simulink model "CoproductReact"  (R2023b)
settings: Solver=VariableStepAuto  StartTime=0.0  StopTime=10.0  RelTol=1e-3
values from neighbouring files (symbols this model uses):
  sug_init = 1011.832    [init_4_sim.m]    (also in init_sim.m = 1011; init_sim2.m; init_sim_suggarferm.m)
  volume = 25    [init_4_sim.m]    (also in init_sim.m; init_sim2.m; init_sim_suggarferm.m)
  yeast_gram = 11    [init_4_sim.m]    (also in init_sim2.m; init_sim_suggarferm.m)
settings Model: Creator=20181234  LastModifiedBy=20181234

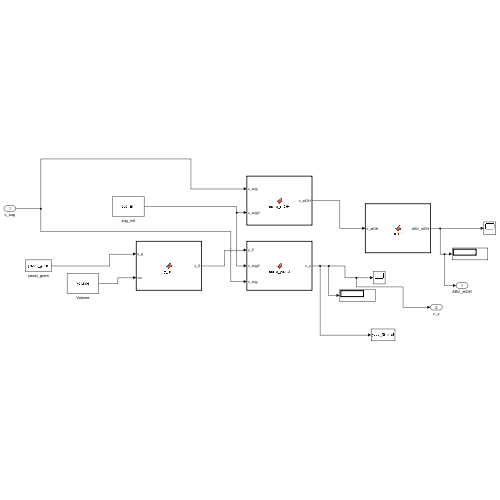
[thumbnail: Simulink's stored preview of the top-level diagram]
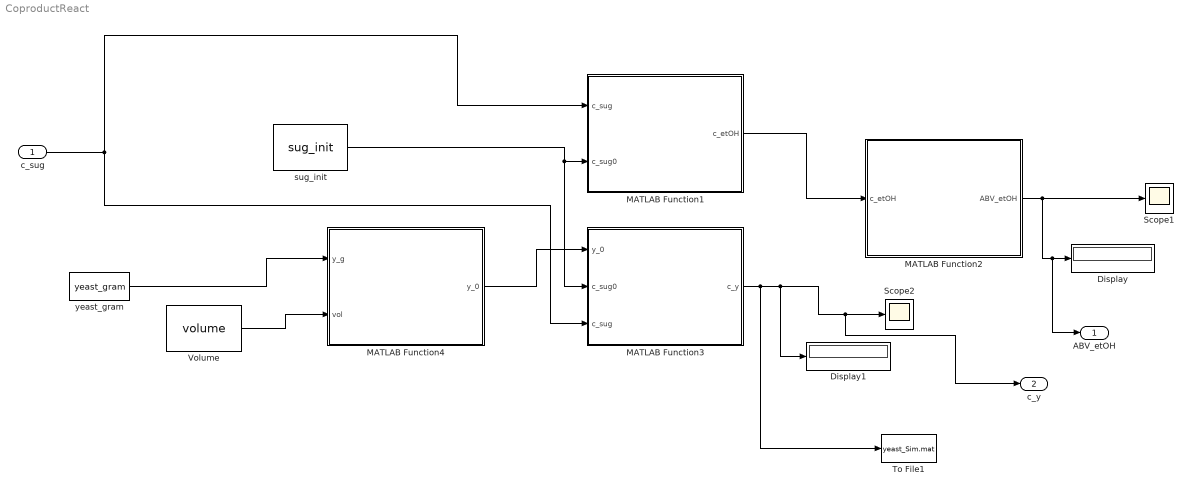
== system CoproductReact ==
  c_sug : Inport
  Display : Display
  Display1 : Display
  MATLAB Function1 : MATLAB Function  TreatAsAtomicUnit=on
  MATLAB Function2 : MATLAB Function  TreatAsAtomicUnit=on
  MATLAB Function3 : MATLAB Function  TreatAsAtomicUnit=on
  MATLAB Function4 : MATLAB Function  TreatAsAtomicUnit=on
  Scope1 : Scope
  Scope2 : Scope
  To File1 : ToFile  Filename=yeast_Sim.mat  MatrixName=yeast
      settings: Decimation=2
  Volume : Constant  Value=volume
  sug_init : Constant  Value=sug_init
  yeast_gram : Constant  Value=yeast_gram
  ABV_etOH : Outport
  c_y : Outport  Port=2
  wires:
  MATLAB Function4/1(y_0) -> MATLAB Function3/1(y_0)
  Volume/1 -> MATLAB Function4/2(vol)
  sug_init/1 -> MATLAB Function3/2(c_sug0), MATLAB Function1/2(c_sug0)
  MATLAB Function3/1(c_y) -> To File1/1, Display1/1, c_y/1, Scope2/1
  yeast_gram/1 -> MATLAB Function4/1(y_g)
  MATLAB Function2/1(ABV_etOH) -> ABV_etOH/1, Display/1, Scope1/1
  MATLAB Function1/1(c_etOH) -> MATLAB Function2/1(c_etOH)
  c_sug/1 -> MATLAB Function3/3(c_sug), MATLAB Function1/1(c_sug)

== matlab function CoproductReact/MATLAB Function1 ==
  data: c_sug input; c_etOH output; c_sug0 input
function c_etOH = conc_etOH(c_sug,c_sug0)
%stequimetry
st= 1.503;
%st= 1.5075;



c_etOH = (c_sug0-c_sug)*st;

== matlab function CoproductReact/MATLAB Function2 ==
  data: c_etOH input; ABV_etOH output
function ABV_etOH = ABV(c_etOH)
%stequimetry
MW_etOH = 46;%mol/g
density_etOH = 0.789; %g/ml




ABV_etOH = c_etOH*(MW_etOH/density_etOH)/1000^2*100;

== matlab function CoproductReact/MATLAB Function3 ==
  data: y_0 input; c_sug0 input; c_sug input; c_y output
function c_y = conc_yeast(y_0,c_sug0,c_sug)
%stequimetry
Y_trans = 0.1;
MW_sug = 180.16; %g/mol
MW_y = 24; %g/mol



c_y = (c_sug0-c_sug)*(MW_sug/MW_y)*Y_trans+y_0;

== matlab function CoproductReact/MATLAB Function4 ==
  data: y_g input; vol input; y_0 output
function y_0 = y_init(y_g,vol)

MW_y = 24; %g/mol


y_0 = (y_g/(vol*1000))/MW_y;
